simulink subsystem "controller_hil"  (R2025b)
settings: Solver=VariableStepAuto  StartTime=0.0  StopTime=10.0  RelTol=1e-3
undefined symbols (not defined in the file or in its folder): dt_control
libraries: ros2lib x2
settings Model: Creator=koryh  LastModifiedBy=vulcangrip

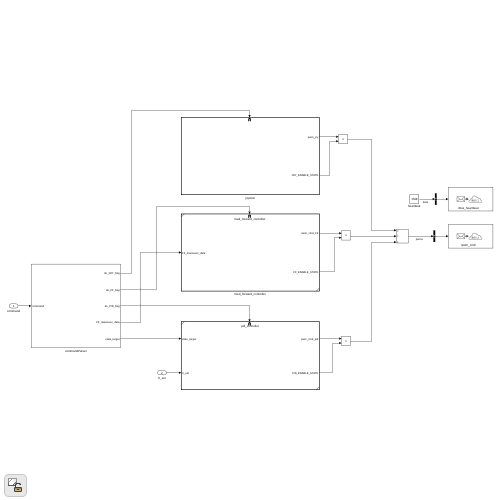
[thumbnail: Simulink's stored preview of the top-level diagram]
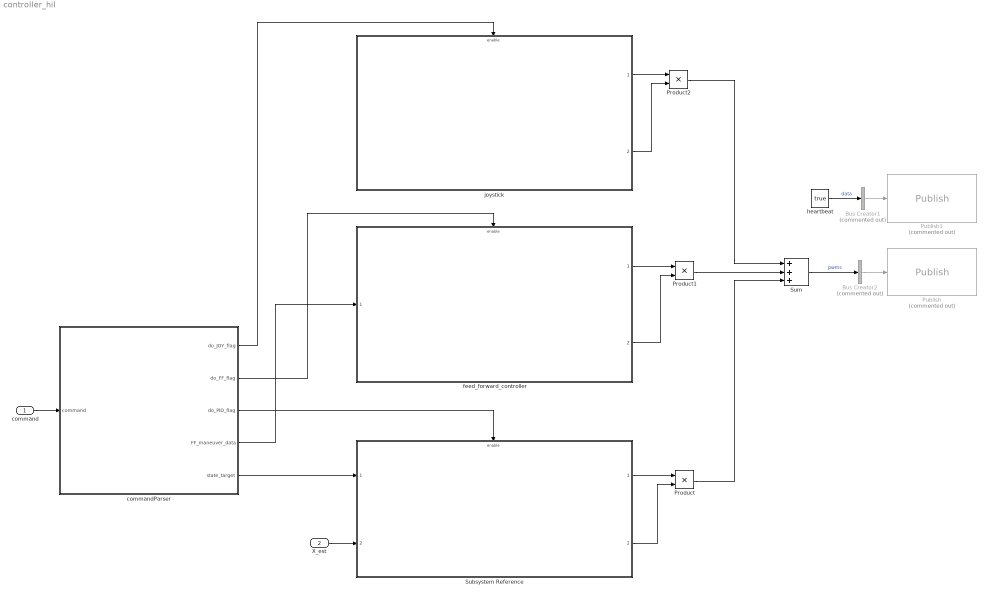
== system controller_hil ==
  command : Inport  SampleTime=dt_control
  X_est : Inport  Port=2  SampleTime=dt_control
  Bus Creator1 : BusCreator  Commented=on  Inputs=1
  Bus Creator2 : BusCreator  Commented=on  Inputs=1  OutDataTypeStr=Bus: SL_Bus_std_msgs_Bool  NonVirtualBus=on
  Product : Product
  Product1 : Product
  Product2 : Product
  Publish : ros2lib/Publish  Commented=on  topicSource=Specify your own  topic=/pwm_cmd  messageType=custom_interfaces/Pwms  QOSHistory=Keep last  QOSDepth=10  QOSReliability=Reliable  QOSDurability=Volatile  QOSDeadline=Inf  QOSLifespan=Inf  QOSLiveliness=Automatic  QOSLeaseDuration=Inf  QOSAvoidROSNamespaceConventions=off
  Publish1 : ros2lib/Publish  Commented=on  topicSource=Specify your own  topic=/mux_heartbeat  messageType=std_msgs/Bool  QOSHistory=Keep last  QOSDepth=10  QOSReliability=Reliable  QOSDurability=Volatile  QOSDeadline=Inf  QOSLifespan=Inf  QOSLiveliness=Automatic  QOSLeaseDuration=Inf  QOSAvoidROSNamespaceConventions=off
  Subsystem Reference : Subsystem  ReferencedSubsystem=pid_controller
  Sum : Sum  Inputs=+|+|+
  commandParser : Subsystem
  feed_forward_controller : Subsystem  ReferencedSubsystem=feed_forward_controller
  heartbeat : Constant  Value=true
  joystick : Subsystem  ReferencedSubsystem=joystick_controller
  wires:
  command/1 -> commandParser/1(command)
  Subsystem Reference/1 -> Product/1
  Subsystem Reference/2 -> Product/2
  commandParser/4(FF_maneuver_data) -> feed_forward_controller/1
  feed_forward_controller/1 -> Product1/1
  feed_forward_controller/2 -> Product1/2
  commandParser/5(state_target) -> Subsystem Reference/1
  X_est/1 -> Subsystem Reference/2
  commandParser/3(do_PID_flag) -> Subsystem Reference/Enable
  heartbeat/1 -> Bus Creator1/1  "data"
  Bus Creator1/1 -> Publish1/1
  Product1/1 -> Sum/2
  Product/1 -> Sum/3
  Sum/1 -> Bus Creator2/1  "pwms"
  Bus Creator2/1 -> Publish/1
  joystick/1 -> Product2/1
  joystick/2 -> Product2/2
  Product2/1 -> Sum/1
  commandParser/2(do_FF_flag) -> feed_forward_controller/Enable
  commandParser/1(do_JOY_flag) -> joystick/Enable

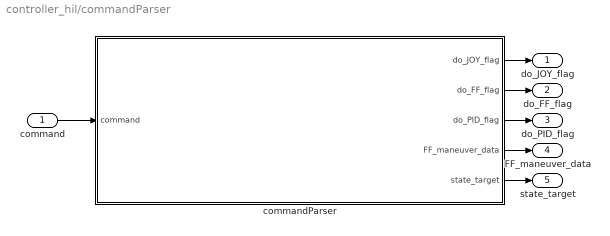
== system controller_hil/commandParser ==
  command : Inport
  commandParser : MATLAB Function  TreatAsAtomicUnit=on
  do_JOY_flag : Outport
  do_FF_flag : Outport  Port=2
  do_PID_flag : Outport  Port=3
  FF_maneuver_data : Outport  Port=4
  state_target : Outport  Port=5
  wires:
  command/1 -> commandParser/1(command)
  commandParser/2(do_FF_flag) -> do_FF_flag/1
  commandParser/3(do_PID_flag) -> do_PID_flag/1
  commandParser/4(FF_maneuver_data) -> FF_maneuver_data/1
  commandParser/5(state_target) -> state_target/1
  commandParser/1(do_JOY_flag) -> do_JOY_flag/1

== matlab function controller_hil/commandParser/commandParser ==
  data: do_JOY_flag output; command input; do_FF_flag output; do_PID_flag output; FF_maneuver_data output; state_target output
function [do_JOY_flag,do_FF_flag,do_PID_flag,FF_maneuver_data,state_target] = fcn(command)

[do_JOY_flag,do_FF_flag,do_PID_flag,FF_maneuver_data,state_target] = commandParser(command);
